simulink model "Modelling_of_Solar_Cell_with_PhotoGenerated_Current_and_Diode_Subsystems"  (R2025a)
settings: Solver=ode23tb  StartTime=0.0  StopTime=2  MaxStep=1e-4  RelTol=1e-3
libraries: simulink x1
settings Model: Creator=Jawad  LastModifiedBy=Jawad
settings DataIOCC: SaveFormat=Array  ReturnWorkspaceOutputs=off

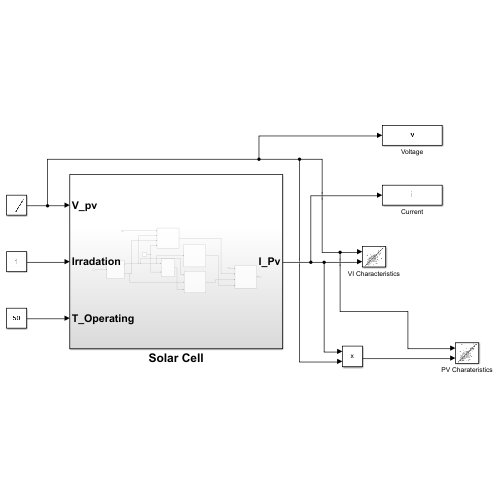
[thumbnail: Simulink's stored preview of the top-level diagram]
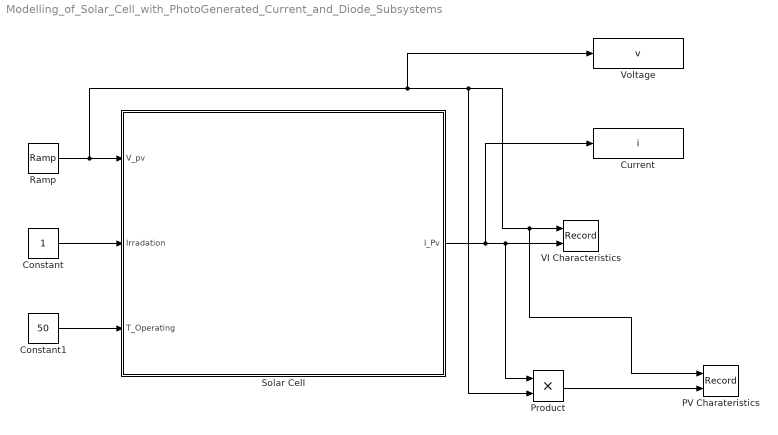
== system Modelling_of_Solar_Cell_with_PhotoGenerated_Current_and_Diode_Subsystems ==
  Constant : Constant
  Constant1 : Constant  Value=50
  Current : ToWorkspace  VariableName=i  SampleTime=-1
  PV Charateristics : Record  NumPorts=2.0  FileSettingsInternal="{\"entries\":[{\"content\":{\"excelSettings\":{\"content\":{},\"type\":\"Streamout.ExcelSettings\"},\"parquetSettings\":{\"content\":{},\"type\":\"Streamout.ParquetSettings\"}},\"type\":\"Streamout.FileSettingStorage\",\"uuid\":\"\"}],\"packageUris\":[\"http:\\/\\/schema.mathworks.com\\/mf0\\/streamout_blocks\\/R2020a\"],\"version\":\"1.0\"}"  FrameSettings=[0, 0]  Layout=[1 2]  SignalsInternal="{\"entries\":[{\"content\":{\"signals\":[{\"content\":{\"blockPath\":[],\"dimensions\":[1],\"domain\":\"\",\"lineColor\":\"#ff6929\",\"lineWidth\":2,\"port\":1,\"sid\":[\"\"],\"signalID\":1,\"signalName\":\"Ramp\"},\"type\":\"RecordBlkView.Signal\",\"uuid\":\"\"},{\"content\":{\"blockPath\":[],\"dimensions\":[1],\"domain\":\"\",\"lineColor\":\"#22b573\",\"lineWidth\":5,\"plots\":[ 1 ],\"port\":2,\"sid\":[\"\"],\"signalID\":2,\"signalName\":\"Product\"},\"type\":\"RecordBlkView.Signal\",\"uuid\":\"\"}]},\"type\":\"RecordBlkView.InputSignals\",\"uuid\":\"\"}],\"packageUris\":[\"http:\\/\\/schema.mathworks.com\\/mf0\\/streamout_blocks\\/R2020a\"],\"version\":\"1.0\"}"  VisualizationBindings="{\"xyplotplugin\":{\"info\":[{\"series\":[{\"bindingParametersList\":[{\"parameter\":\"Y-Axis\",\"signalID\":2,\"signalName\":\"Product\"}],\"seriesID\":0}],\"subplotID\":1}]}}"  CompatibilityTag=XY
  Product : Product
  Ramp : simulink/Sources/Ramp  slope=22  start=0  InitialOutput=0
  Solar Cell : Subsystem
  VI Characteristics : Record  NumPorts=2.0  FileSettingsInternal="{\"entries\":[{\"content\":{\"excelSettings\":{\"content\":{},\"type\":\"Streamout.ExcelSettings\"},\"parquetSettings\":{\"content\":{},\"type\":\"Streamout.ParquetSettings\"}},\"type\":\"Streamout.FileSettingStorage\",\"uuid\":\"\"}],\"packageUris\":[\"http:\\/\\/schema.mathworks.com\\/mf0\\/streamout_blocks\\/R2020a\"],\"version\":\"1.0\"}"  FrameSettings=[0, 0]  Layout=[1 1]  SignalsInternal="{\"entries\":[{\"content\":{\"signals\":[{\"content\":{\"blockPath\":[],\"dimensions\":[1],\"domain\":\"\",\"lineColor\":\"#64d413\",\"lineWidth\":2,\"port\":1,\"sid\":[\"\"],\"signalID\":1,\"signalName\":\"Ramp\"},\"type\":\"RecordBlkView.Signal\",\"uuid\":\"\"},{\"content\":{\"blockPath\":[],\"dimensions\":[1],\"domain\":\"\",\"lineColor\":\"#ff13a6\",\"lineWidth\":2,\"port\":2,\"sid\":[\"\"],\"signalID\":2,\"signalName\":\"Solar Cell\"},\"type\":\"RecordBlkView.Signal\",\"uuid\":\"\"}]},\"type\":\"RecordBlkView.InputSignals\",\"uuid\":\"\"}],\"packageUris\":[\"http:\\/\\/schema.mathworks.com\\/mf0\\/streamout_blocks\\/R2020a\"],\"version\":\"1.0\"}"  VisualizationBindings="{\"xyplotplugin\":{\"info\":[{\"series\":[],\"subplotID\":1}]}}"  CompatibilityTag=XY
  Voltage : ToWorkspace  VariableName=v  SampleTime=-1
  wires:
  Ramp/1 -> Voltage/1, Product/2, PV Charateristics/1, VI Characteristics/1, Solar Cell/1(V_pv)
  Constant/1 -> Solar Cell/2(Irradation)
  Constant1/1 -> Solar Cell/3(T_Operating)
  Solar Cell/1(I_Pv) -> Current/1, Product/1, VI Characteristics/2
  Product/1 -> PV Charateristics/2

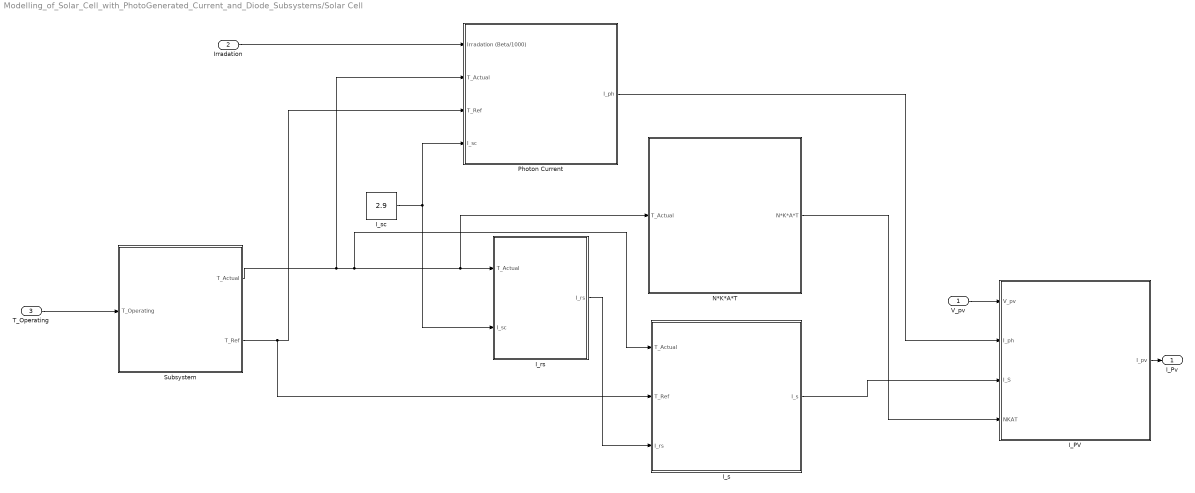
== system Modelling_of_Solar_Cell_with_PhotoGenerated_Current_and_Diode_Subsystems/Solar Cell ==
  V_pv : Inport
  Irradation : Inport  Port=2
  T_Operating : Inport  Port=3
  I_PV : Subsystem
  I_rs : Subsystem
  I_s : Subsystem
  I_sc : Constant  Value=2.9
  N*K*A*T : Subsystem
  Photon Current : Subsystem
  Subsystem : Subsystem
  I_Pv : Outport
  wires:
  N*K*A*T/1(N*K*A*T) -> I_PV/4(NKAT)
  I_rs/1(I_rs) -> I_s/3(I_rs)
  T_Operating/1 -> Subsystem/1(T_Operating)
  Subsystem/1(T_Actual) -> Photon Current/2(T_Actual), I_s/1(T_Actual), N*K*A*T/1(T_Actual), I_rs/1(T_Actual)
  Subsystem/2(T_Ref) -> I_s/2(T_Ref), Photon Current/3(T_Ref)
  V_pv/1 -> I_PV/1(V_pv)
  Irradation/1 -> Photon Current/1(Irradation (Beta/1000))
  I_sc/1 -> I_rs/2(I_sc), Photon Current/4(I_sc)
  Photon Current/1(I_ph) -> I_PV/2(I_ph)
  I_s/1(I_s) -> I_PV/3(I_S)
  I_PV/1(I_pv) -> I_Pv/1

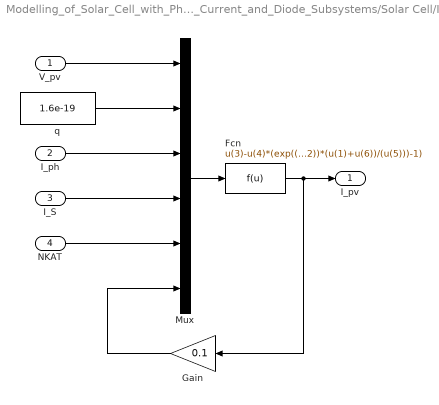
== system Modelling_of_Solar_Cell_with_PhotoGenerated_Current_and_Diode_Subsystems/Solar Cell/I_PV ==
  V_pv : Inport
  I_ph : Inport  Port=2
  I_S : Inport  Port=3
  NKAT : Inport  Port=4
  Fcn : Fcn  Expr=u(3)-u(4)*(exp((u(2))*(u(1)+u(6))/(u(5)))-1)
  Gain : Gain  Gain=0.1
  Mux : Mux  Inputs=6
  q : Constant  Value=1.6e-19
  I_pv : Outport
  wires:
  Gain/1 -> Mux/6
  Fcn/1 -> I_pv/1, Gain/1
  NKAT/1 -> Mux/5
  I_ph/1 -> Mux/3
  I_S/1 -> Mux/4
  V_pv/1 -> Mux/1
  Mux/1 -> Fcn/1
  q/1 -> Mux/2

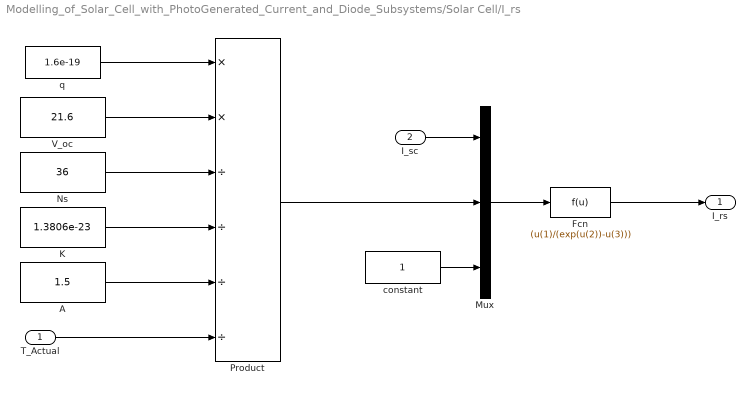
== system Modelling_of_Solar_Cell_with_PhotoGenerated_Current_and_Diode_Subsystems/Solar Cell/I_rs ==
  T_Actual : Inport
  I_sc : Inport  Port=2
  A : Constant  Value=1.5
  Fcn : Fcn  Expr=(u(1)/(exp(u(2))-u(3)))
  K : Constant  Value=1.3806e-23
  Mux : Mux  Inputs=3
  Ns : Constant  Value=36
  Product : Product  Inputs=**////
  V_oc : Constant  Value=21.6
  constant : Constant
  q : Constant  Value=1.6e-19
  I_rs : Outport
  wires:
  q/1 -> Product/1
  K/1 -> Product/4
  T_Actual/1 -> Product/6
  I_sc/1 -> Mux/1
  Product/1 -> Mux/2
  Mux/1 -> Fcn/1
  V_oc/1 -> Product/2
  Ns/1 -> Product/3
  constant/1 -> Mux/3
  A/1 -> Product/5
  Fcn/1 -> I_rs/1

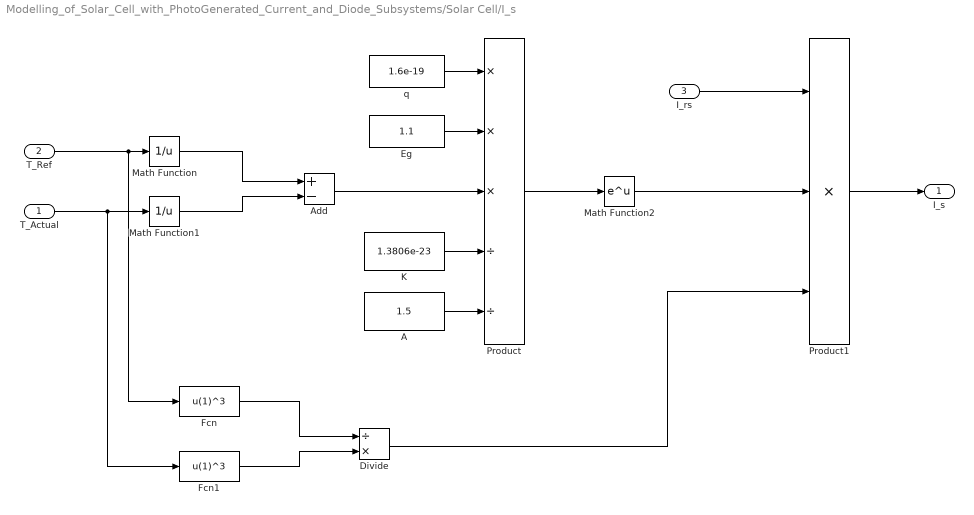
== system Modelling_of_Solar_Cell_with_PhotoGenerated_Current_and_Diode_Subsystems/Solar Cell/I_s ==
  T_Actual : Inport
  T_Ref : Inport  Port=2
  I_rs : Inport  Port=3
  A : Constant  Value=1.5
  Add : Sum  Inputs=+-
  Divide : Product  Inputs=/*
  Eg : Constant  Value=1.1
  Fcn : Fcn  Expr=u(1)^3
  Fcn1 : Fcn  Expr=u(1)^3
  K : Constant  Value=1.3806e-23
  Math Function : Math  Operator=reciprocal
  Math Function1 : Math  Operator=reciprocal
  Math Function2 : Math
  Product : Product  Inputs=***//
  Product1 : Product  Inputs=***
  q : Constant  Value=1.6e-19
  I_s : Outport
  wires:
  K/1 -> Product/4
  q/1 -> Product/1
  Eg/1 -> Product/2
  T_Ref/1 -> Fcn/1, Math Function/1
  Math Function/1 -> Add/1
  T_Actual/1 -> Fcn1/1, Math Function1/1
  A/1 -> Product/5
  Product/1 -> Math Function2/1
  Divide/1 -> Product1/3
  Fcn1/1 -> Divide/2
  Add/1 -> Product/3
  Math Function1/1 -> Add/2
  I_rs/1 -> Product1/1
  Math Function2/1 -> Product1/2
  Fcn/1 -> Divide/1
  Product1/1 -> I_s/1

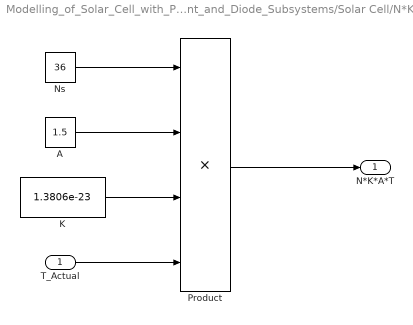
== system Modelling_of_Solar_Cell_with_PhotoGenerated_Current_and_Diode_Subsystems/Solar Cell/N*K*A*T ==
  T_Actual : Inport
  A : Constant  Value=1.5
  K : Constant  Value=1.3806e-23
  Ns : Constant  Value=36
  Product : Product  Inputs=4
  N*K*A*T : Outport
  wires:
  Product/1 -> N*K*A*T/1
  Ns/1 -> Product/1
  T_Actual/1 -> Product/4
  K/1 -> Product/3
  A/1 -> Product/2

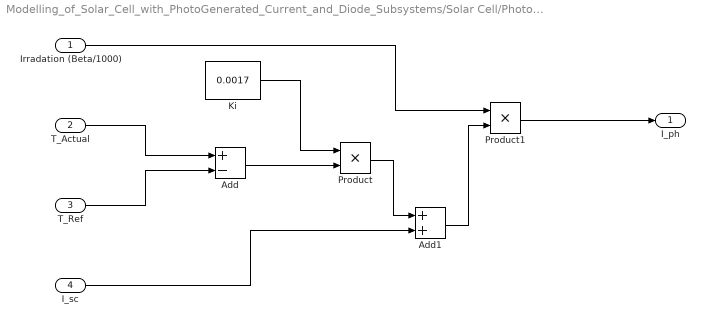
== system Modelling_of_Solar_Cell_with_PhotoGenerated_Current_and_Diode_Subsystems/Solar Cell/Photon Current ==
  Irradation (Beta/1000) : Inport
  T_Actual : Inport  Port=2
  T_Ref : Inport  Port=3
  I_sc : Inport  Port=4
  Add : Sum  Inputs=+-
  Add1 : Sum
  Ki : Constant  Value=0.0017
  Product : Product
  Product1 : Product
  I_ph : Outport
  wires:
  Product1/1 -> I_ph/1
  I_sc/1 -> Add1/2
  T_Actual/1 -> Add/1
  Add1/1 -> Product1/2
  T_Ref/1 -> Add/2
  Product/1 -> Add1/1
  Irradation (Beta/1000)/1 -> Product1/1
  Ki/1 -> Product/1
  Add/1 -> Product/2

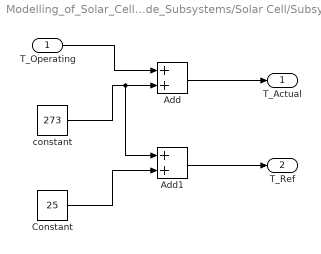
== system Modelling_of_Solar_Cell_with_PhotoGenerated_Current_and_Diode_Subsystems/Solar Cell/Subsystem ==
  T_Operating : Inport
  Add : Sum
  Add1 : Sum
  Constant : Constant  Value=25
  constant : Constant  Value=273
  T_Actual : Outport
  T_Ref : Outport  Port=2
  wires:
  constant/1 -> Add1/1, Add/2
  T_Operating/1 -> Add/1
  Add/1 -> T_Actual/1
  Constant/1 -> Add1/2
  Add1/1 -> T_Ref/1
